simulink model "switch"  (R2014a)
settings: Solver=ode3  StartTime=0.0  StopTime=10.0  FixedStep=0.1  RelTol=1e-3
libraries: simulink x1
settings Model: Creator=eruffaldi  LastModifiedBy=eruffaldi

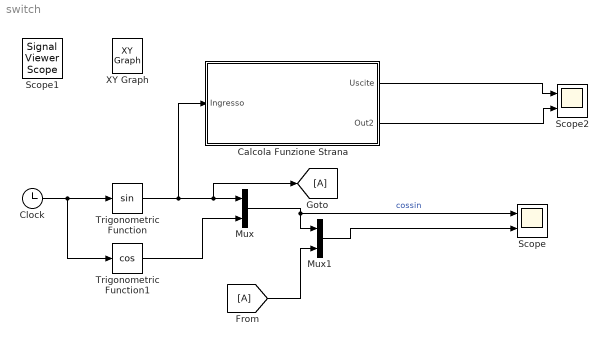
== system switch ==
  Calcola Funzione Strana : Subsystem
  Clock : Clock
  Mux : Mux  Inputs=2
  Mux1 : Mux  Inputs=2
  Scope : Scope  NumInputPorts=2
      settings: TimeRange=10  YMin=-1~-1  YMax=1~1
  Scope2 : Scope  NumInputPorts=2
      settings: TimeRange=10  YMin=-1~-1  YMax=1~1
  Trigonometric Function : Trigonometry
  Trigonometric Function1 : Trigonometry  Operator=cos
  Scope1 : SignalViewerScope  IOType=viewer  RefreshTime=0.035000
  XY Graph : simulink/Sinks/XY Graph  IOType=viewer  xmin=-1  xmax=1  ymin=-1  ymax=1  st=-1
  wires:
  Clock/1 -> Trigonometric Function1/1, Trigonometric Function/1
  Trigonometric Function/1 -> Calcola Funzione Strana/1(Ingresso), [A], Mux/1
  Trigonometric Function1/1 -> Mux/2
  Mux/1 -> Mux1/1, Scope/1  "cossin"
  Mux1/1 -> Scope/2
  [A] -> Mux1/2
  Calcola Funzione Strana/1(Uscite) -> Scope2/1
  Calcola Funzione Strana/2(Out2) -> Scope2/2

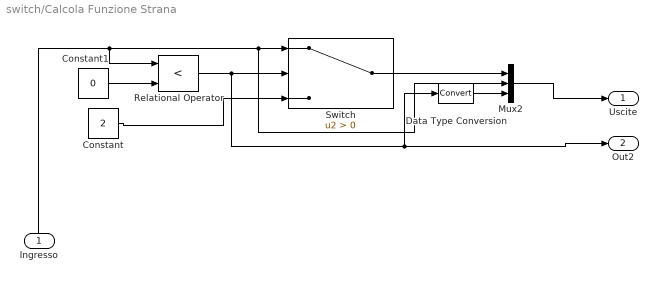
== system switch/Calcola Funzione Strana ==
  Ingresso : Inport
  Constant : Constant  Value=2
  Constant1 : Constant  Value=0
  Data Type Conversion : DataTypeConversion
  Mux2 : Mux  Inputs=3
  Relational Operator : RelationalOperator  Operator=<  OutDataTypeStr=boolean
  Switch : Switch  Criteria=u2 > Threshold
  Uscite : Outport
  Out2 : Outport  Port=2
  wires:
  Relational Operator/1 -> Out2/1, Data Type Conversion/1, Switch/2
  Switch/1 -> Mux2/1
  Mux2/1 -> Uscite/1
  Constant/1 -> Switch/3
  Ingresso/1 -> Relational Operator/1, Mux2/2, Switch/1
  Constant1/1 -> Relational Operator/2
  Data Type Conversion/1 -> Mux2/3
